simulink model "modello_controllore3"  (R2025a)
settings: Solver=ode45  StartTime=0.0  StopTime=10  FixedStep=0.001  RelTol=1e-7  AbsTol=1e-9
values from neighbouring files (symbols this model uses):
  K = 1004.096    [closed_loop_identification_frequency.m]
  M = 2.010    (= 2.01)    [closed_loop_identification_frequency.m]    (also in stima_senza_simulink.m = P.M)
  Mm = 1.0036    [closed_loop_identification_frequency.m]    (also in stima_senza_simulink.m = P.Mm)
undefined symbols (not defined in the file or in its folder): Kd_tau, Kd_theta, Kp_tau, Kp_theta
settings Model: Creator=hp  LastModifiedBy=riccardodaguanno
settings DataIOCC: SaveFormat=StructureWithTime  SaveOutput=off

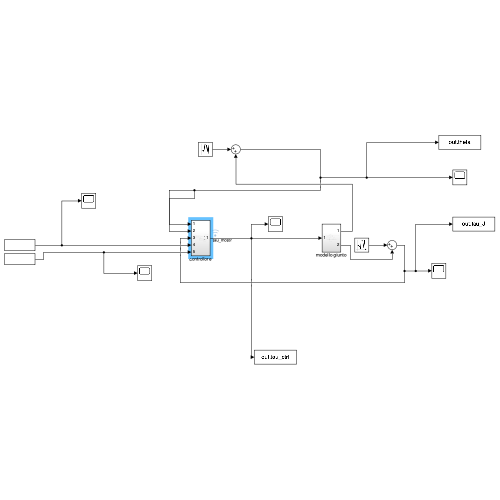
[thumbnail: Simulink's stored preview of the top-level diagram]
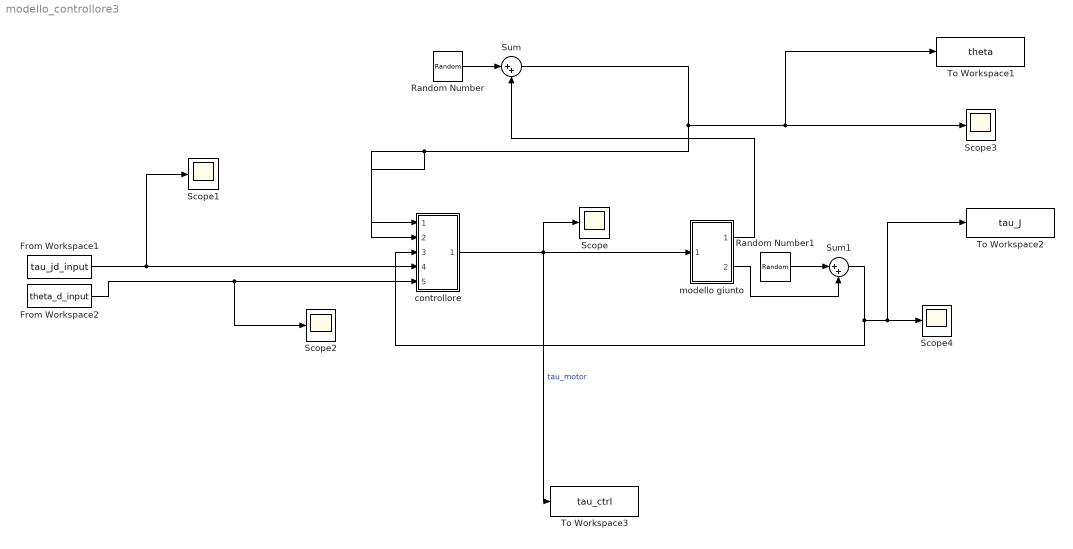
== system modello_controllore3 ==
  From Workspace1 : FromWorkspace  VariableName=tau_jd_input  OutputAfterFinalValue=Holding final value
  From Workspace2 : FromWorkspace  VariableName=theta_d_input  OutputAfterFinalValue=Holding final value
  Random Number : RandomNumber  Variance=0  SampleTime=0.001
  Random Number1 : RandomNumber  Variance=0  SampleTime=0.001
  Scope{,1..4} (5 alike) : Scope
      Scope settings: ActiveDisplayYMinimum=-346.7950077033837  ActiveDisplayYMaximum=329.83772179817618  DataLoggingVariableName=ScopeData5
      Scope1 settings: ActiveDisplayYMinimum=-1  ActiveDisplayYMaximum=1  DataLoggingVariableName=ScopeData6
      Scope2 settings: ActiveDisplayYMinimum=-1  ActiveDisplayYMaximum=1  DataLoggingVariableName=ScopeData7
      Scope3 settings: ActiveDisplayYMinimum=-11.562827971819823  ActiveDisplayYMaximum=16.890529809572982  DataLoggingVariableName=ScopeData8
      Scope4 settings: ActiveDisplayYMinimum=-6.07092860920146E+14  ActiveDisplayYMaximum=2.020941359764075E+15  DataLoggingVariableName=ScopeData9
  Sum : Sum  Inputs=|++
  Sum1 : Sum  Inputs=|++
  To Workspace1 : ToWorkspace  VariableName=theta  SaveFormat=Timeseries  SampleTime=-1
  To Workspace2 : ToWorkspace  VariableName=tau_J  SaveFormat=Timeseries  SampleTime=-1
  To Workspace3 : ToWorkspace  VariableName=tau_ctrl  SaveFormat=Timeseries  SampleTime=-1
  controllore : Subsystem
  modello giunto : Subsystem
  wires:
  controllore/1(Out1) -> To Workspace3/1, modello giunto/1(In1), Scope/1  "tau_motor"
  From Workspace1/1 -> Scope1/1, controllore/4(In4)
  From Workspace2/1 -> Scope2/1, controllore/5(In5)
  Random Number/1 -> Sum/1
  modello giunto/1(Out1) -> Sum/2
  Sum/1 -> controllore/2(In2), controllore/1(In1), To Workspace1/1, Scope3/1
  Random Number1/1 -> Sum1/1
  Sum1/1 -> controllore/3(In3), To Workspace2/1, Scope4/1
  modello giunto/2(Out2) -> Sum1/2

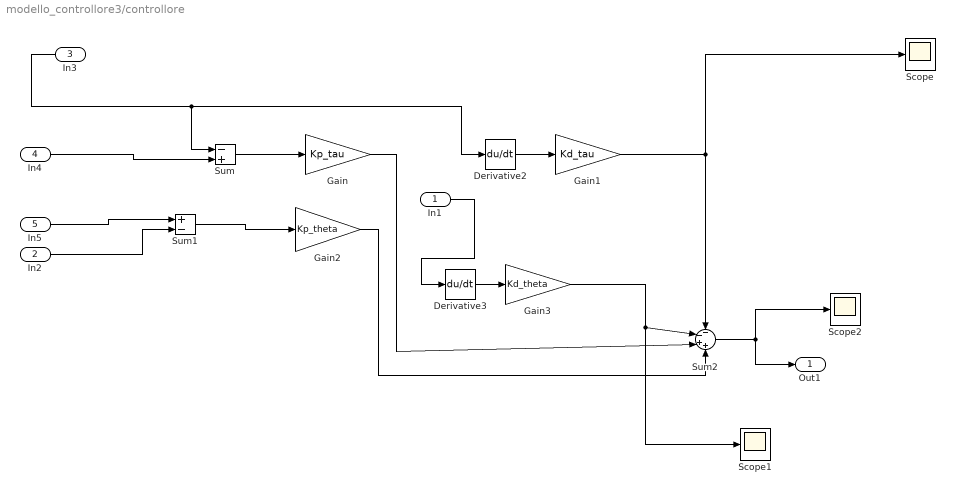
== system modello_controllore3/controllore ==
  In1 : Inport
  In2 : Inport  Port=2
  In3 : Inport  Port=3
  In4 : Inport  Port=4
  In5 : Inport  Port=5
  Derivative2 : Derivative
  Derivative3 : Derivative
  Gain : Gain  Gain=Kp_tau
  Gain1 : Gain  Gain=Kd_tau
  Gain2 : Gain  Gain=Kp_theta
  Gain3 : Gain  Gain=Kd_theta
  Scope : Scope
      settings: ActiveDisplayYMinimum=-6371.606522150747  ActiveDisplayYMaximum=5822.552631567678  DataLoggingVariableName=ScopeData3
  Scope1 : Scope
      settings: ActiveDisplayYMinimum=-60.078386734880489  ActiveDisplayYMaximum=96.298420272429112  DataLoggingVariableName=ScopeData4
  Scope2 : Scope
      settings: ActiveDisplayYMinimum=-1867.9248565799312  ActiveDisplayYMaximum=2405.0224937241392  DataLoggingVariableName=ScopeData10
  Sum : Sum  Inputs=-+
  Sum1 : Sum  Inputs=+-
  Sum2 : Sum  Inputs=--++
  Out1 : Outport
  wires:
  In1/1 -> Derivative3/1
  In2/1 -> Sum1/2
  In5/1 -> Sum1/1
  Sum1/1 -> Gain2/1
  Gain1/1 -> Scope/1, Sum2/1
  Sum/1 -> Gain/1
  In3/1 -> Derivative2/1, Sum/1
  Gain2/1 -> Sum2/4
  Gain/1 -> Sum2/3
  Sum2/1 -> Scope2/1, Out1/1
  In4/1 -> Sum/2
  Gain3/1 -> Scope1/1, Sum2/2
  Derivative2/1 -> Gain1/1
  Derivative3/1 -> Gain3/1

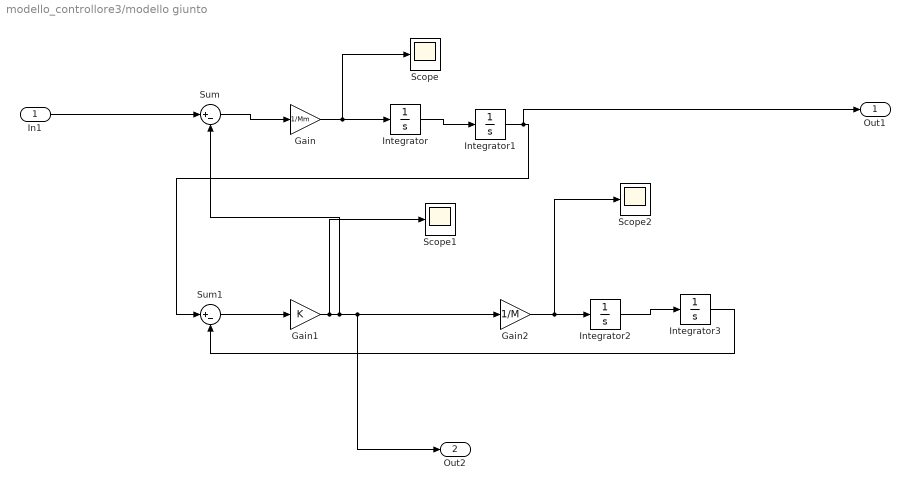
== system modello_controllore3/modello giunto ==
  In1 : Inport
  Gain : Gain  Gain=1/Mm
  Gain1 : Gain  Gain=K
  Gain2 : Gain  Gain=1/M
  Integrator{,1..3} (4 alike) : Integrator
  Scope : Scope
      settings: ActiveDisplayYMinimum=-11.120378605520472  ActiveDisplayYMaximum=53.660873476191959
  Scope1 : Scope
      settings: ActiveDisplayYMinimum=-9.8963676788809423  ActiveDisplayYMaximum=10.00811088374217
  Scope2 : Scope
      settings: ActiveDisplayYMinimum=-3.76702  ActiveDisplayYMaximum=4.09748  DataLoggingVariableName=ScopeData2
  Sum : Sum  Inputs=|+-
  Sum1 : Sum  Inputs=|+-
  Out1 : Outport
  Out2 : Outport  Port=2
  wires:
  In1/1 -> Sum/1
  Gain/1 -> Scope/1, Integrator/1
  Integrator2/1 -> Integrator3/1
  Sum/1 -> Gain/1
  Integrator1/1 -> Out1/1, Sum1/1
  Integrator3/1 -> Sum1/2
  Sum1/1 -> Gain1/1
  Integrator/1 -> Integrator1/1
  Gain1/1 -> Scope1/1, Sum/2, Out2/1, Gain2/1
  Gain2/1 -> Scope2/1, Integrator2/1
